simulink model "deadzone_nonlinearity"  (R2024a)
settings: Solver=FixedStepAuto  StartTime=0.0  StopTime=7.5  FixedStep=1e-6  RelTol=1e-3
libraries: simulink x1
settings Model: Creator=Lenovo  LastModifiedBy=Lenovo

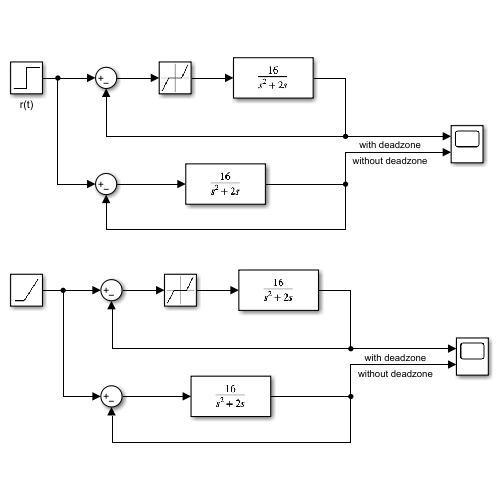
[thumbnail: Simulink's stored preview of the top-level diagram]
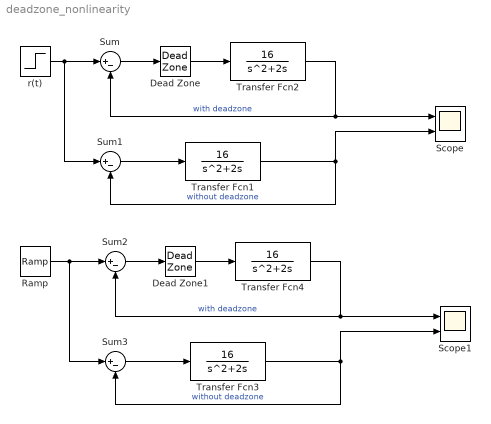
== system deadzone_nonlinearity ==
  Dead Zone : DeadZone  LowerValue=-0.2  UpperValue=0.2
  Dead Zone1 : DeadZone  LowerValue=-0.2  UpperValue=0.2
  Ramp : simulink/Sources/Ramp  slope=2  start=0  InitialOutput=0
  Scope : Scope  NumInputPorts=2
  Scope1 : Scope  NumInputPorts=2
  Sum{,1..3} (4 alike) : Sum  Inputs=|+-
  Transfer Fcn{1..4} (4 alike) : TransferFcn  Numerator=[16]  Denominator=[1 2 0]
  r(t) : Step  Time=0  SampleTime=0
  wires:
  r(t)/1 -> Sum1/1, Sum/1
  Dead Zone/1 -> Transfer Fcn2/1
  Transfer Fcn1/1 -> Sum1/2, Scope/2  "without deadzone"
  Sum1/1 -> Transfer Fcn1/1
  Sum/1 -> Dead Zone/1
  Transfer Fcn2/1 -> Scope/1, Sum/2  "with deadzone"
  Transfer Fcn4/1 -> Sum2/2, Scope1/1  "with deadzone"
  Sum2/1 -> Dead Zone1/1
  Sum3/1 -> Transfer Fcn3/1
  Transfer Fcn3/1 -> Scope1/2, Sum3/2  "without deadzone"
  Dead Zone1/1 -> Transfer Fcn4/1
  Ramp/1 -> Sum2/1, Sum3/1
